simulink model "balon_model"  (Simulink 7.7)
settings: Solver=ode45  StartTime=0.0  StopTime=40000  RelTol=1e-3
values from neighbouring files (symbols this model uses):
  Cd = 0.5    [s1.m]
  Cw = 1005    [s1.m]
  g = 9.80665    [s1.m]
  Gmz = G * mz    (= 398345073000000)    [s1.m]
  kWymianyCiepla = 0.5    [s1.m]
  mb = 113.4 + 63.5 + 22.7 + 183.7 + 340.2    (= 723.5)    [s1.m]
  Mp = 0.028970    (= 0.02897)    [s1.m]
  P = 2000000    [s1.m]
  p0 = 101325    [s1.m]
  Ppb = 3.1415 * (19/2)^2    (= 283.520375)    [s1.m]
  promienZiemii = 6360000    [s1.m]
  R = 8.314    [s1.m]
  ro0 = 1.2250    (= 1.225)    [s1.m]
  spadekTemp = 0.0065    [s1.m]
  sprP = 0.08    [s1.m]
  T0 = 273.15 + 20    (= 293.15)    [s1.m]
  V = 2800    [s1.m]
settings Model: Creator=Jakub  LastModifiedBy=Jakub
settings SolverCC: AlgebraicLoopSolver=LineSearch

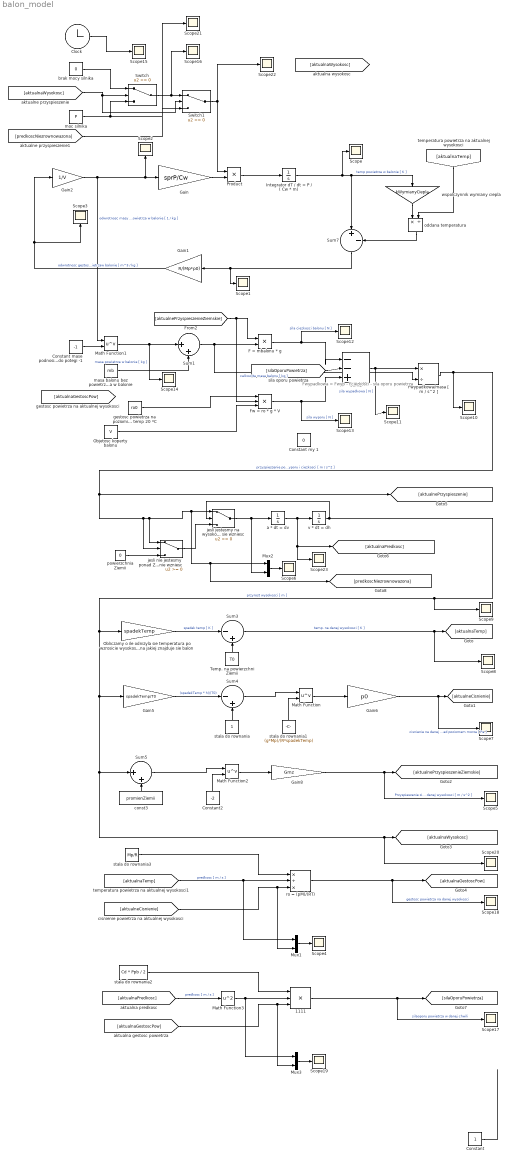
== system balon_model ==
  note: Fwypadkowa =
      | Fwyp - Fciezkosci
      | - sila oporu powietrza
  1111 : Product  Inputs=***  RndMeth=Zero
  Clock : Clock
      settings: Decimation=10
  Constant : Constant
  Constant mase podnosimy  do potegi -1 : Constant  Value=-1
  Constant my 1 : Constant  Value=0
  Constant2 : Constant  Value=-2
  F = mbalonu * g : Product  RndMeth=Zero
  Fw = ro * g * V : Product  Inputs=3  RndMeth=Zero
  Fwypadkowa/masa [ m / s^2 ] : Product  Inputs=*/  RndMeth=Zero
  Gain : Gain  Gain=sprP/Cw
  Gain1 : Gain  Gain=R/(Mp*p0)
  Gain2 : Gain  Gain=1/V
  Gain5 : Gain  Gain=spadekTemp/T0
  Gain6 : Gain  Gain=p0
  Gain8 : Gain  Gain=Gmz
  Integrator dT / dt = P / ( Cw * m) : Integrator  InitialCondition=T0
  Math Function : Math  Operator=pow  SaturateOnIntegerOverflow=on
  Math Function1 : Math  Operator=pow  SaturateOnIntegerOverflow=on
  Math Function2 : Math  Operator=pow  SaturateOnIntegerOverflow=on
  Math Function3 : Math  Operator=square  SaturateOnIntegerOverflow=on
  Mux1 : Mux  Inputs=2
  Mux2 : Mux  Inputs=2
  Mux3 : Mux  Inputs=2
  Objetosc koperty balonu : Constant  Value=V
  Obliczamy o ile odnizyla sie temperatura po wzrosicie wysokosci na jakiej znajduje sie balon : Gain  Gain=spadekTemp
  Product : Product  RndMeth=Zero
  Scope{,1..23} (24 alike) : Scope
      Scope10 settings: SaveName=ScopeData10
      Scope11 settings: SaveName=ScopeData11
      Scope12 settings: SaveName=ScopeData12
      Scope13 settings: SaveName=ScopeData13
      Scope14 settings: SaveName=ScopeData14
      Scope15 settings: SaveName=ScopeData15
      Scope16 settings: SaveName=ScopeData16
      Scope17 settings: SaveName=ScopeData17
      Scope18 settings: SaveName=ScopeData18
      Scope19 settings: SaveName=ScopeData19
      Scope2 settings: SaveName=ScopeData2
      Scope20 settings: SaveName=ScopeData20
      Scope21 settings: SaveName=ScopeData21
      Scope22 settings: SaveName=ScopeData22
      Scope23 settings: YMin=0.06  YMax=0.0975  SaveName=ScopeData23
      Scope3 settings: SaveName=ScopeData3
      Scope4 settings: SaveName=ScopeData4
      Scope5 settings: SaveName=ScopeData5
      Scope6 settings: YMin=0.06  YMax=0.0975  SaveName=ScopeData6
      Scope7 settings: SaveName=ScopeData7
      Scope8 settings: SaveName=ScopeData8
      Scope9 settings: YMin=0.004575  YMax=0.0049  SaveName=ScopeData9
  Sum1 : Sum  Inputs=|++
  Sum2 : Sum  Inputs=|--+
  Sum3 : Sum  Inputs=|-+
  Sum4 : Sum  Inputs=|-+
  Sum5 : Sum  Inputs=|++
  Sum7 : Sum  Inputs=|+-
  Switch : Switch
  Switch1 : Switch
  Temp. na powierzchni Ziemii : Constant  Value=T0
  a * dt = dv : Integrator
  brak mocy silnika : Constant  Value=0
  const3 : Constant  Value=promienZiemii
  gestosc powietrza na poziomie morza przy  temp 20 *C : Constant  Value=ro0
  "jesli jestesmy na wysokosci dodatniej, to mozemy opasc lub sie wzniesc" : Switch
  jesli nie jestesmy ponad Ziemia to mozemy sie jedynie wzniesc : Switch
  masa balonu bez powietrza w balonie : Constant  Value=mb
  moc silnika : Constant  Value=P
  oddana temperatura : Product  Inputs=*/  RndMeth=Zero
  powierzchnia Ziemii : Constant  Value=0
  ro = (pM)/(RT) : Product  Inputs=*/*  RndMeth=Zero
  stala do rownania : Constant
  stala do rownania1 : Constant  Value=(g*Mp)/(R*spadekTemp)
  stala do rownania2 : Constant  Value=Cd * Ppb / 2
  stala do rownania3 : Constant  Value=Mp/R
  v * dt = dh : Integrator
  wspolczynnik wymiany ciepla : Gain  Gain=kWymianyCiepla
  wires:
  Integrator dT / dt = P / ( Cw * m)/1 -> Scope/1, Sum7/1, wspolczynnik wymiany ciepla/1  "temp powietrza w balonie [ K ]"
  Gain1/1 -> Gain2/1, Scope3/1  "odwrotnosc gestosci  powietrzaw balonie [ m^3 / kg ]"
  Gain2/1 -> Gain/1, Scope2/1, Math Function1/1  "odwrotnosc masy powietrza w balonie [ 1 / kg ]"
  Constant mase podnosimy  do potegi -1/1 -> Math Function1/2
  Math Function1/1 -> Sum1/1, Scope14/1  "masa powietrza w balonie [ kg ]"
  masa balonu bez powietrza w balonie/1 -> Sum1/2
  Sum1/1 -> F = mbalonu * g/2, Fwypadkowa/masa [ m / s^2 ]/2  "calkowita masa balonu [ kg ]"
  [aktualnePrzyspieszenieZiemskie] -> F = mbalonu * g/1, Fw = ro * g * V/2
  F = mbalonu * g/1 -> Sum2/1, Scope12/1  "sila ciezkosci balonu [ N ]"
  Objetosc koperty balonu/1 -> Fw = ro * g * V/3
  Fw = ro * g * V/1 -> Scope13/1, Sum2/3  "sila wyporu [ N ]"
  Sum2/1 -> Fwypadkowa/masa [ m / s^2 ]/1, Scope11/1  "sila wypadkowa [ N ]"
  Fwypadkowa/masa [ m / s^2 ]/1 -> Scope10/1, [aktualnePrzyspieszenie], jesli nie jestesmy ponad Ziemia to mozemy sie jedynie wzniesc/2, jesli nie jestesmy ponad Ziemia to mozemy sie jedynie wzniesc/1, "jesli jestesmy na wysokosci dodatniej, to mozemy opasc lub sie wzniesc"/1, Mux2/1, [predkoscNiezrownowazona]  "przyspieszenie powstale w wyniku sily wyporu i ciezkosci [ m / s^2 ]"
  v * dt = dh/1 -> "jesli jestesmy na wysokosci dodatniej, to mozemy opasc lub sie wzniesc"/2, Obliczamy o ile odnizyla sie temperatura po wzrosicie wysokosci na jakiej znajduje sie balon/1, Gain5/1, Sum5/1, [aktualnaWysokosc], Scope20/1, Scope9/1  "przyrost wysokosci [ m ]"
  "jesli jestesmy na wysokosci dodatniej, to mozemy opasc lub sie wzniesc"/1 -> a * dt = dv/1, Mux2/2
  jesli nie jestesmy ponad Ziemia to mozemy sie jedynie wzniesc/1 -> "jesli jestesmy na wysokosci dodatniej, to mozemy opasc lub sie wzniesc"/3
  powierzchnia Ziemii/1 -> jesli nie jestesmy ponad Ziemia to mozemy sie jedynie wzniesc/3
  Mux2/1 -> Scope6/1
  Temp. na powierzchni Ziemii/1 -> Sum3/2
  Obliczamy o ile odnizyla sie temperatura po wzrosicie wysokosci na jakiej znajduje sie balon/1 -> Sum3/1  "spadek temp [ K ]"
  Sum3/1 -> [aktualnaTemp], Scope8/1  "temp. na danej wysokosci [ K ]"
  Gain5/1 -> Sum4/1  "(spadekTemp * h)/(T0)"
  stala do rownania/1 -> Sum4/2
  Sum4/1 -> Math Function/1
  stala do rownania1/1 -> Math Function/2
  Math Function/1 -> Gain6/1
  Gain6/1 -> [aktualneCisnienie], Scope7/1  "cisnienie na danej wysokosci nad poziomem morza [ Pa ]"
  const3/1 -> Sum5/2
  Sum5/1 -> Math Function2/1
  Constant2/1 -> Math Function2/2
  Math Function2/1 -> Gain8/1
  Gain8/1 -> [aktualnePrzyspieszenieZiemskie], Scope5/1  "Przyspieszenie ziemskie na danej wysokosci [ m / s^2 ]"
  Constant/1 -> ?
  Sum7/1 -> Gain1/1, Scope1/1
  oddana temperatura/1 -> Sum7/2
  wspolczynnik wymiany ciepla/1 -> oddana temperatura/1
  [aktualnaTemp] -> oddana temperatura/2
  stala do rownania3/1 -> ro = (pM)/(RT)/1
  [aktualneCisnienie] -> ro = (pM)/(RT)/3, Mux1/2
  [aktualnaTemp] -> ro = (pM)/(RT)/2, Mux1/1  "predkosc [ m / s ]"
  ro = (pM)/(RT)/1 -> Scope18/1, [aktualnaGestoscPow]  "gestosc powietrza na danej wysokosci"
  Mux1/1 -> Scope4/1
  Clock/1 -> Scope15/1
  brak mocy silnika/1 -> Switch/1
  moc silnika/1 -> Switch/3, Switch1/3
  Product/1 -> Integrator dT / dt = P / ( Cw * m)/1
  Gain/1 -> Product/2
  Switch/1 -> Scope16/1, Switch1/1
  gestosc powietrza na poziomie morza przy  temp 20 *C/1 -> Fw = ro * g * V/1
  stala do rownania2/1 -> 1111/1
  [aktualnaGestoscPow] -> 1111/3, Mux3/2
  [aktualnaPredkosc] -> Math Function3/1  "predkosc [ m / s ]"
  1111/1 -> Scope17/1, [silaOporuPowietrza]  "silaoporu powietrza w danej chwili"
  Mux3/1 -> Scope19/1
  Math Function3/1 -> 1111/2, Mux3/1
  [silaOporuPowietrza] -> Sum2/2
  Switch1/1 -> Product/1, Scope22/1
  [predkoscNiezrownowazona] -> Scope21/1
  a * dt = dv/1 -> v * dt = dh/1, [aktualnaPredkosc], Scope23/1
  [aktualnaWysokosc] -> Switch/2, Switch1/2
